simulink model "test_sys2"  (R2013b)
settings: Solver=ode45  StartTime=0.0  StopTime=5000  RelTol=1e-3
undefined symbols (not defined in the file or in its folder): twiddle_factors, xlipgetpartsetting
libraries: xbsIndex_r4 x2526, casper_library_misc x201, xps_library x1
(part 1 of 29)
settings Model: Creator=root  LastModifiedBy=root

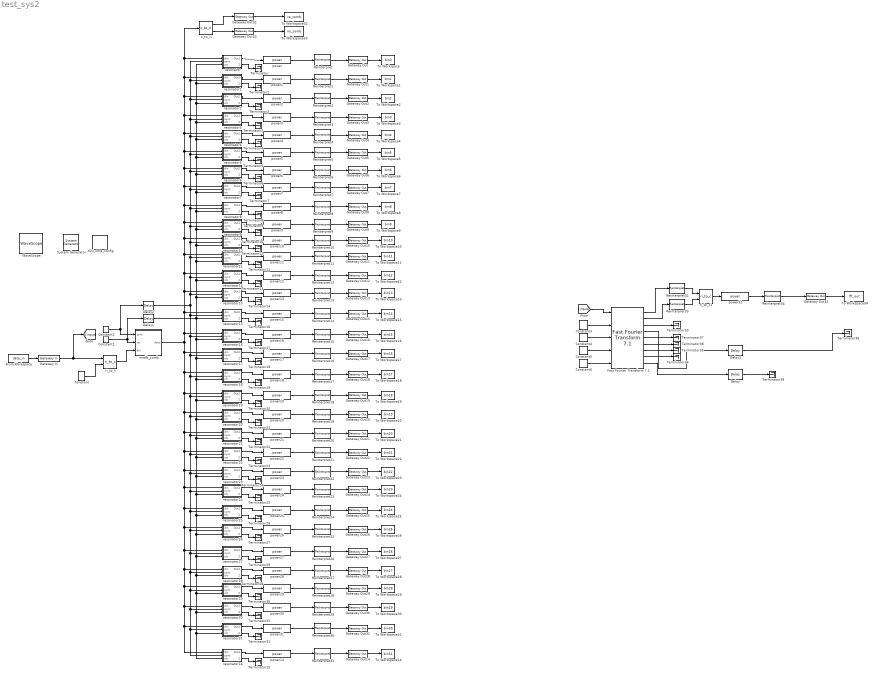
== system test_sys2 ==
  " System Generator" : xbsIndex_r4/ System Generator  Tag=genX  xilinxfamily=Kintex7  part=xc7k325t  speed=-3  package=fbg676  synthesis_tool=XST  clock_wrapper=Clock Enables  directory=./netlist  proj_type=Project Navigator  Synth_file=XST Defaults  Impl_file=ISE Defaults  testbench=off  simulink_period=1  sysclk_period=10  dcm_input_clock_period=10  incr_netlist=off  trim_vbits=Everywhere in SubSystem  dbl_ovrd=According to Block Masks  core_generation=According to Block Masks  run_coregen=off  deprecated_control=off  eval_field=0  block_type=sysgen
  Constant : xbsIndex_r4/Constant  const=0  gui_display_data_type=Fixed-point  arith_type=Signed (2's comp)  n_bits=10  bin_pt=9  preci_type=Single  exp_width=8  frac_width=24  explicit_period=on  period=1  equ=P=C  opselect=C  inp2=PCIN>>17  opr=+  inp1=P  carry=CIN  dbl_ovrd=off  block_type=constant
  Constant1 : xbsIndex_r4/Constant  const=0  gui_display_data_type=Boolean  arith_type=Boolean  n_bits=16  bin_pt=14  preci_type=Single  exp_width=8  frac_width=24  explicit_period=on  period=1  equ=P=C  opselect=C  inp2=PCIN>>17  opr=+  inp1=P  carry=CIN  dbl_ovrd=off  block_type=constant
  Constant2 : xbsIndex_r4/Constant  const=1  gui_display_data_type=Boolean  arith_type=Boolean  n_bits=16  bin_pt=14  preci_type=Single  exp_width=8  frac_width=24  explicit_period=on  period=1  equ=P=C  opselect=C  inp2=PCIN>>17  opr=+  inp1=P  carry=CIN  dbl_ovrd=off  block_type=constant
  Constant3 : xbsIndex_r4/Constant  const=0  gui_display_data_type=Fixed-point  arith_type=Signed (2's comp)  n_bits=10  bin_pt=9  preci_type=Single  exp_width=8  frac_width=24  explicit_period=on  period=1  equ=P=C  opselect=C  inp2=PCIN>>17  opr=+  inp1=P  carry=CIN  dbl_ovrd=off  block_type=constant
  Constant4 : xbsIndex_r4/Constant  const=1  gui_display_data_type=Boolean  arith_type=Boolean  n_bits=10  bin_pt=9  preci_type=Single  exp_width=8  frac_width=24  explicit_period=on  period=1  equ=P=C  opselect=C  inp2=PCIN>>17  opr=+  inp1=P  carry=CIN  dbl_ovrd=off  block_type=constant
  Constant5 : xbsIndex_r4/Constant  const=1  gui_display_data_type=Boolean  arith_type=Boolean  n_bits=10  bin_pt=9  preci_type=Single  exp_width=8  frac_width=24  explicit_period=on  period=1  equ=P=C  opselect=C  inp2=PCIN>>17  opr=+  inp1=P  carry=CIN  dbl_ovrd=off  block_type=constant
  Constant6 : xbsIndex_r4/Constant  const=0  gui_display_data_type=Boolean  arith_type=Boolean  n_bits=10  bin_pt=9  preci_type=Single  exp_width=8  frac_width=24  explicit_period=on  period=1  equ=P=C  opselect=C  inp2=PCIN>>17  opr=+  inp1=P  carry=CIN  dbl_ovrd=off  block_type=constant
  Delay : xbsIndex_r4/Delay  rst=off  infoeditControl=Selection of Reset will increase slice count due to use of real FFs and instead of SRLs  en=off  latency=5  dbl_ovrd=off  reg_retiming=off  block_type=delay
  Delay1 : xbsIndex_r4/Delay  rst=off  infoeditControl=Selection of Reset will increase slice count due to use of real FFs and instead of SRLs  en=off  latency=1  dbl_ovrd=off  reg_retiming=off  block_type=delay
  Delay2 : xbsIndex_r4/Delay  rst=off  infoeditControl=Selection of Reset will increase slice count due to use of real FFs and instead of SRLs  en=off  latency=1  dbl_ovrd=off  reg_retiming=off  block_type=delay
  Delay3 : xbsIndex_r4/Delay  rst=off  infoeditControl=Selection of Reset will increase slice count due to use of real FFs and instead of SRLs  en=off  latency=5  dbl_ovrd=off  reg_retiming=off  block_type=delay
  "Fast Fourier Transform 7.1 " : xbsIndex_r4/Fast Fourier Transform 7.1   transform_length=128  implementation_options=pipelined_streaming_io  target_clock_frequency=250  target_data_throughput=50  run_time_configurable_transform_length=off  phase_factor_width=16  scaling_options=unscaled  rounding_modes=convergent_rounding  output_ordering=natural_order  cyclic_prefix_insertion=off  ce=off  sclr=off  ovflo=off  input_data_offset=three_cycle_offset  memory_options_data=block_ram  memory_options_phase_factors=block_ram  number_of_stages_using_block_ram_for_data_and_phase_factors=1  memory_options_reorder=block_ram  memory_options_hybrid=off  complex_mult_type=use_mults_performance  butterfly_type=use_luts  channels=1  input_ordering=natural_order  input_width=16  simulation_type=external_xfix  simulation_model=fftv71_CModel:fftv71_cmodel  ip_name=Fast Fourier Transform  ip_version=7.1  dsptool_ready=true  wrapper_available=true  port_translation_map={ 'ce' => 'en', 'sclr' => 'rst' }  ipcore_fpga_part=xlipgetpartsetting(gcb, {'virtex4', 'xc4vsx35', '-10', 'ff668'})  block_type=xfft_v7_1
  From Workspace : FromWorkspace  VariableName=data_in  SampleTime=0
  Gateway In : xbsIndex_r4/Gateway In  gui_display_data_type=Fixed-point  arith_type="Signed  (2's comp)"  n_bits=10  bin_pt=9  preci_type=Single  exp_width=8  frac_width=24  quantization="Round  (unbiased: +/- Inf)"  overflow=Saturate  period=1  dbl_ovrd=off  timing_constraint=None  locs_specified=off  LOCs={}  UseAsADC=off  ADCChannel='1'  inherit_from_input=off  hdl_port=on  block_type=gatewayin
  Gateway Out{,1..34} (35 alike) : xbsIndex_r4/Gateway Out  inherit_from_input=off  hdl_port=on  timing_constraint=None  locs_specified=off  LOCs={}  UseAsDAC=off  DACChannel='1'  block_type=gatewayout
  Reinterpret{,1..31,34} (33 alike) : xbsIndex_r4/Reinterpret  force_arith_type=off  arith_type=Unsigned  force_bin_pt=on  bin_pt=0  block_type=reinterpret
  Reinterpret32 : xbsIndex_r4/Reinterpret  force_arith_type=off  arith_type=Unsigned  force_bin_pt=on  bin_pt=17  block_type=reinterpret
  Reinterpret33 : xbsIndex_r4/Reinterpret  force_arith_type=off  arith_type=Unsigned  force_bin_pt=on  bin_pt=17  block_type=reinterpret
  Terminator{,1..39} (40 alike) : Terminator
  To Workspace : ToWorkspace  VariableName=bin0  SampleTime=-1  SaveFormat=Timeseries
  To Workspace1 : ToWorkspace  VariableName=bin1  SampleTime=-1  SaveFormat=Timeseries
  To Workspace10 : ToWorkspace  VariableName=bin10  SampleTime=-1  SaveFormat=Timeseries
  To Workspace11 : ToWorkspace  VariableName=bin11  SampleTime=-1  SaveFormat=Timeseries
  To Workspace12 : ToWorkspace  VariableName=bin12  SampleTime=-1  SaveFormat=Timeseries
  To Workspace13 : ToWorkspace  VariableName=bin13  SampleTime=-1  SaveFormat=Timeseries
  To Workspace14 : ToWorkspace  VariableName=bin31  SampleTime=-1  SaveFormat=Timeseries
  To Workspace15 : ToWorkspace  VariableName=bin14  SampleTime=-1  SaveFormat=Timeseries
  To Workspace16 : ToWorkspace  VariableName=bin15  SampleTime=-1  SaveFormat=Timeseries
  To Workspace17 : ToWorkspace  VariableName=bin16  SampleTime=-1  SaveFormat=Timeseries
  To Workspace18 : ToWorkspace  VariableName=bin17  SampleTime=-1  SaveFormat=Timeseries
  To Workspace19 : ToWorkspace  VariableName=bin18  SampleTime=-1  SaveFormat=Timeseries
  To Workspace2 : ToWorkspace  VariableName=bin2  SampleTime=-1  SaveFormat=Timeseries
  To Workspace20 : ToWorkspace  VariableName=bin19  SampleTime=-1  SaveFormat=Timeseries
  To Workspace21 : ToWorkspace  VariableName=bin20  SampleTime=-1  SaveFormat=Timeseries
  To Workspace22 : ToWorkspace  VariableName=bin21  SampleTime=-1  SaveFormat=Timeseries
  To Workspace23 : ToWorkspace  VariableName=bin22  SampleTime=-1  SaveFormat=Timeseries
  To Workspace24 : ToWorkspace  VariableName=bin23  SampleTime=-1  SaveFormat=Timeseries
  To Workspace25 : ToWorkspace  VariableName=bin24  SampleTime=-1  SaveFormat=Timeseries
  To Workspace26 : ToWorkspace  VariableName=bin25  SampleTime=-1  SaveFormat=Timeseries
  To Workspace27 : ToWorkspace  VariableName=bin26  SampleTime=-1  SaveFormat=Timeseries
  To Workspace28 : ToWorkspace  VariableName=bin27  SampleTime=-1  SaveFormat=Timeseries
  To Workspace29 : ToWorkspace  VariableName=bin28  SampleTime=-1  SaveFormat=Timeseries
  To Workspace3 : ToWorkspace  VariableName=bin3  SampleTime=-1  SaveFormat=Timeseries
  To Workspace30 : ToWorkspace  VariableName=bin29  SampleTime=-1  SaveFormat=Timeseries
  To Workspace31 : ToWorkspace  VariableName=bin30  SampleTime=-1  SaveFormat=Timeseries
  To Workspace32 : ToWorkspace  VariableName=re_comb  SampleTime=-1  SaveFormat=Timeseries
  To Workspace33 : ToWorkspace  VariableName=im_comb  SampleTime=-1  SaveFormat=Timeseries
  To Workspace34 : ToWorkspace  VariableName=fft_out  SampleTime=-1  SaveFormat=Timeseries
  To Workspace4 : ToWorkspace  VariableName=bin4  SampleTime=-1  SaveFormat=Timeseries
  To Workspace5 : ToWorkspace  VariableName=bin5  SampleTime=-1  SaveFormat=Timeseries
  To Workspace6 : ToWorkspace  VariableName=bin6  SampleTime=-1  SaveFormat=Timeseries
  To Workspace7 : ToWorkspace  VariableName=bin7  SampleTime=-1  SaveFormat=Timeseries
  To Workspace8 : ToWorkspace  VariableName=bin8  SampleTime=-1  SaveFormat=Timeseries
  To Workspace9 : ToWorkspace  VariableName=bin9  SampleTime=-1  SaveFormat=Timeseries
  WaveScope : xbsIndex_r4/WaveScope  block_type=wavescope
  XSG_core_config : xps_library/XSG_core_config  Tag=xps:xsg  hw_sys=ROACH2:sx475t  clk_src=sys_clk  ROACH_clk_src=sys_clk  ROACH2_clk_src=sys_clk  MKDIG_clk_src=sys_clk  clk_rate=100  sample_period=1  synthesis_tool=XST
  c_to_ri : casper_library_misc/c_to_ri  n_bits=11  bin_pt=9
      settings: AttributesFormatString=11_9 r/i
  msdft_comb : Subsystem  mask(msdft_comb){input_bitsize=10, fft_len=7, latency=0}
      mask prompts: fft_len "fft_len (2^?)"; latency "sub latency"
      mask init:
      | msdft_comb_init(gcb, ...
      |         'input_bitsize', input_bitsize, ...
      |         'fft_len', fft_len, ...
      |         'latency', latency);
      settings: AttributesFormatString=latency=0
  power{,1..31} (32 alike) : casper_library_misc/power  BitWidth=40  add_latency=2  mult_latency=3
  power32 : casper_library_misc/power  BitWidth=18  add_latency=2  mult_latency=3
  resonator : Subsystem  mask(msdft_res){fft_len=7, twid_bitsize=15, bin_number=0, input_bitsize=11, input_frac=9, res_bitsize=40, add_lat=0}
      mask prompts: fft_len "fft len(2^?)"; twid_bitsize "twid bitsize"; bin_number "bin number"; input_bitsize "input bitsize"; input_frac "input frac"; res_bitsize "out resonator size"
      mask init:
      | msdft_resonator_init(gcb, ...
      |                 'fft_len', fft_len, ...
      |                 'twid_bitsize', twid_bitsize, ...
      |                 'bin_number', bin_number, ...
      |                 'input_bitsize', input_bitsize, ...
      |                 'input_frac', input_frac, ...
      |                 'res_bitsize', res_bitsize, ...
      |                 'add_lat', add_lat);
      settings: AttributesFormatString=N=7, k=0
  resonator1 : Subsystem  mask(msdft_res){fft_len=7, twid_bitsize=15, bin_number=1, input_bitsize=11, input_frac=9, res_bitsize=40, add_lat=0}
      mask prompts: fft_len "fft len(2^?)"; twid_bitsize "twid bitsize"; bin_number "bin number"; input_bitsize "input bitsize"; input_frac "input frac"; res_bitsize "out resonator size"
      mask init: same as test_sys2/resonator
      settings: AttributesFormatString=N=7, k=1
  resonator10 : Subsystem  mask(msdft_res){fft_len=7, twid_bitsize=15, bin_number=10, input_bitsize=11, input_frac=9, res_bitsize=40, add_lat=0}
      mask prompts: fft_len "fft len(2^?)"; twid_bitsize "twid bitsize"; bin_number "bin number"; input_bitsize "input bitsize"; input_frac "input frac"; res_bitsize "out resonator size"
      mask init: same as test_sys2/resonator
      settings: AttributesFormatString=N=7, k=10
  resonator11 : Subsystem  mask(msdft_res){fft_len=7, twid_bitsize=15, bin_number=11, input_bitsize=11, input_frac=9, res_bitsize=40, add_lat=0}
      mask prompts: fft_len "fft len(2^?)"; twid_bitsize "twid bitsize"; bin_number "bin number"; input_bitsize "input bitsize"; input_frac "input frac"; res_bitsize "out resonator size"
      mask init: same as test_sys2/resonator
      settings: AttributesFormatString=N=7, k=11
  resonator12 : Subsystem  mask(msdft_res){fft_len=7, twid_bitsize=15, bin_number=12, input_bitsize=11, input_frac=9, res_bitsize=40, add_lat=0}
      mask prompts: fft_len "fft len(2^?)"; twid_bitsize "twid bitsize"; bin_number "bin number"; input_bitsize "input bitsize"; input_frac "input frac"; res_bitsize "out resonator size"
      mask init: same as test_sys2/resonator
      settings: AttributesFormatString=N=7, k=12
  resonator13 : Subsystem  mask(msdft_res){fft_len=7, twid_bitsize=15, bin_number=13, input_bitsize=11, input_frac=9, res_bitsize=40, add_lat=0}
      mask prompts: fft_len "fft len(2^?)"; twid_bitsize "twid bitsize"; bin_number "bin number"; input_bitsize "input bitsize"; input_frac "input frac"; res_bitsize "out resonator size"
      mask init: same as test_sys2/resonator
      settings: AttributesFormatString=N=7, k=13
  resonator14 : Subsystem  mask(msdft_res){fft_len=7, twid_bitsize=15, bin_number=31, input_bitsize=11, input_frac=9, res_bitsize=40, add_lat=0}
      mask prompts: fft_len "fft len(2^?)"; twid_bitsize "twid bitsize"; bin_number "bin number"; input_bitsize "input bitsize"; input_frac "input frac"; res_bitsize "out resonator size"
      mask init: same as test_sys2/resonator
      settings: AttributesFormatString=N=7, k=31
  resonator15 : Subsystem  mask(msdft_res){fft_len=7, twid_bitsize=15, bin_number=14, input_bitsize=11, input_frac=9, res_bitsize=40, add_lat=0}
      mask prompts: fft_len "fft len(2^?)"; twid_bitsize "twid bitsize"; bin_number "bin number"; input_bitsize "input bitsize"; input_frac "input frac"; res_bitsize "out resonator size"
      mask init: same as test_sys2/resonator
      settings: AttributesFormatString=N=7, k=14
  resonator16 : Subsystem  mask(msdft_res){fft_len=7, twid_bitsize=15, bin_number=15, input_bitsize=11, input_frac=9, res_bitsize=40, add_lat=0}
      mask prompts: fft_len "fft len(2^?)"; twid_bitsize "twid bitsize"; bin_number "bin number"; input_bitsize "input bitsize"; input_frac "input frac"; res_bitsize "out resonator size"
      mask init: same as test_sys2/resonator
      settings: AttributesFormatString=N=7, k=15
  resonator17 : Subsystem  mask(msdft_res){fft_len=7, twid_bitsize=15, bin_number=16, input_bitsize=11, input_frac=9, res_bitsize=40, add_lat=0}
      mask prompts: fft_len "fft len(2^?)"; twid_bitsize "twid bitsize"; bin_number "bin number"; input_bitsize "input bitsize"; input_frac "input frac"; res_bitsize "out resonator size"
      mask init: same as test_sys2/resonator
      settings: AttributesFormatString=N=7, k=16
  resonator18 : Subsystem  mask(msdft_res){fft_len=7, twid_bitsize=15, bin_number=17, input_bitsize=11, input_frac=9, res_bitsize=40, add_lat=0}
      mask prompts: fft_len "fft len(2^?)"; twid_bitsize "twid bitsize"; bin_number "bin number"; input_bitsize "input bitsize"; input_frac "input frac"; res_bitsize "out resonator size"
      mask init: same as test_sys2/resonator
      settings: AttributesFormatString=N=7, k=17
  resonator19 : Subsystem  mask(msdft_res){fft_len=7, twid_bitsize=15, bin_number=18, input_bitsize=11, input_frac=9, res_bitsize=40, add_lat=0}
      mask prompts: fft_len "fft len(2^?)"; twid_bitsize "twid bitsize"; bin_number "bin number"; input_bitsize "input bitsize"; input_frac "input frac"; res_bitsize "out resonator size"
      mask init: same as test_sys2/resonator
      settings: AttributesFormatString=N=7, k=18
  resonator2 : Subsystem  mask(msdft_res){fft_len=7, twid_bitsize=15, bin_number=2, input_bitsize=11, input_frac=9, res_bitsize=40, add_lat=0}
      mask prompts: fft_len "fft len(2^?)"; twid_bitsize "twid bitsize"; bin_number "bin number"; input_bitsize "input bitsize"; input_frac "input frac"; res_bitsize "out resonator size"
      mask init: same as test_sys2/resonator
      settings: AttributesFormatString=N=7, k=2
  resonator20 : Subsystem  mask(msdft_res){fft_len=7, twid_bitsize=15, bin_number=19, input_bitsize=11, input_frac=9, res_bitsize=40, add_lat=0}
      mask prompts: fft_len "fft len(2^?)"; twid_bitsize "twid bitsize"; bin_number "bin number"; input_bitsize "input bitsize"; input_frac "input frac"; res_bitsize "out resonator size"
      mask init: same as test_sys2/resonator
      settings: AttributesFormatString=N=7, k=19
  resonator21 : Subsystem  mask(msdft_res){fft_len=7, twid_bitsize=15, bin_number=20, input_bitsize=11, input_frac=9, res_bitsize=40, add_lat=0}
      mask prompts: fft_len "fft len(2^?)"; twid_bitsize "twid bitsize"; bin_number "bin number"; input_bitsize "input bitsize"; input_frac "input frac"; res_bitsize "out resonator size"
      mask init: same as test_sys2/resonator
      settings: AttributesFormatString=N=7, k=20
  resonator22 : Subsystem  mask(msdft_res){fft_len=7, twid_bitsize=15, bin_number=21, input_bitsize=11, input_frac=9, res_bitsize=40, add_lat=0}
      mask prompts: fft_len "fft len(2^?)"; twid_bitsize "twid bitsize"; bin_number "bin number"; input_bitsize "input bitsize"; input_frac "input frac"; res_bitsize "out resonator size"
      mask init: same as test_sys2/resonator
      settings: AttributesFormatString=N=7, k=21
  resonator23 : Subsystem  mask(msdft_res){fft_len=7, twid_bitsize=15, bin_number=22, input_bitsize=11, input_frac=9, res_bitsize=40, add_lat=0}
      mask prompts: fft_len "fft len(2^?)"; twid_bitsize "twid bitsize"; bin_number "bin number"; input_bitsize "input bitsize"; input_frac "input frac"; res_bitsize "out resonator size"
      mask init: same as test_sys2/resonator
      settings: AttributesFormatString=N=7, k=22
  resonator24 : Subsystem  mask(msdft_res){fft_len=7, twid_bitsize=15, bin_number=23, input_bitsize=11, input_frac=9, res_bitsize=40, add_lat=0}
      mask prompts: fft_len "fft len(2^?)"; twid_bitsize "twid bitsize"; bin_number "bin number"; input_bitsize "input bitsize"; input_frac "input frac"; res_bitsize "out resonator size"
      mask init: same as test_sys2/resonator
      settings: AttributesFormatString=N=7, k=23
  resonator25 : Subsystem  mask(msdft_res){fft_len=7, twid_bitsize=15, bin_number=24, input_bitsize=11, input_frac=9, res_bitsize=40, add_lat=0}
      mask prompts: fft_len "fft len(2^?)"; twid_bitsize "twid bitsize"; bin_number "bin number"; input_bitsize "input bitsize"; input_frac "input frac"; res_bitsize "out resonator size"
      mask init: same as test_sys2/resonator
      settings: AttributesFormatString=N=7, k=24
  resonator26 : Subsystem  mask(msdft_res){fft_len=7, twid_bitsize=15, bin_number=25, input_bitsize=11, input_frac=9, res_bitsize=40, add_lat=0}
      mask prompts: fft_len "fft len(2^?)"; twid_bitsize "twid bitsize"; bin_number "bin number"; input_bitsize "input bitsize"; input_frac "input frac"; res_bitsize "out resonator size"
      mask init: same as test_sys2/resonator
      settings: AttributesFormatString=N=7, k=25
  resonator27 : Subsystem  mask(msdft_res){fft_len=7, twid_bitsize=15, bin_number=26, input_bitsize=11, input_frac=9, res_bitsize=40, add_lat=0}
      mask prompts: fft_len "fft len(2^?)"; twid_bitsize "twid bitsize"; bin_number "bin number"; input_bitsize "input bitsize"; input_frac "input frac"; res_bitsize "out resonator size"
      mask init: same as test_sys2/resonator
      settings: AttributesFormatString=N=7, k=26
  resonator28 : Subsystem  mask(msdft_res){fft_len=7, twid_bitsize=15, bin_number=27, input_bitsize=11, input_frac=9, res_bitsize=40, add_lat=0}
      mask prompts: fft_len "fft len(2^?)"; twid_bitsize "twid bitsize"; bin_number "bin number"; input_bitsize "input bitsize"; input_frac "input frac"; res_bitsize "out resonator size"
      mask init: same as test_sys2/resonator
      settings: AttributesFormatString=N=7, k=27
  resonator29 : Subsystem  mask(msdft_res){fft_len=7, twid_bitsize=15, bin_number=28, input_bitsize=11, input_frac=9, res_bitsize=40, add_lat=0}
      mask prompts: fft_len "fft len(2^?)"; twid_bitsize "twid bitsize"; bin_number "bin number"; input_bitsize "input bitsize"; input_frac "input frac"; res_bitsize "out resonator size"
      mask init: same as test_sys2/resonator
      settings: AttributesFormatString=N=7, k=28
  resonator3 : Subsystem  mask(msdft_res){fft_len=7, twid_bitsize=15, bin_number=3, input_bitsize=11, input_frac=9, res_bitsize=40, add_lat=0}
      mask prompts: fft_len "fft len(2^?)"; twid_bitsize "twid bitsize"; bin_number "bin number"; input_bitsize "input bitsize"; input_frac "input frac"; res_bitsize "out resonator size"
      mask init: same as test_sys2/resonator
      settings: AttributesFormatString=N=7, k=3
  resonator30 : Subsystem  mask(msdft_res){fft_len=7, twid_bitsize=15, bin_number=29, input_bitsize=11, input_frac=9, res_bitsize=40, add_lat=0}
      mask prompts: fft_len "fft len(2^?)"; twid_bitsize "twid bitsize"; bin_number "bin number"; input_bitsize "input bitsize"; input_frac "input frac"; res_bitsize "out resonator size"
      mask init: same as test_sys2/resonator
      settings: AttributesFormatString=N=7, k=29
  resonator31 : Subsystem  mask(msdft_res){fft_len=7, twid_bitsize=15, bin_number=30, input_bitsize=11, input_frac=9, res_bitsize=40, add_lat=0}
      mask prompts: fft_len "fft len(2^?)"; twid_bitsize "twid bitsize"; bin_number "bin number"; input_bitsize "input bitsize"; input_frac "input frac"; res_bitsize "out resonator size"
      mask init: same as test_sys2/resonator
      settings: AttributesFormatString=N=7, k=30
  resonator4 : Subsystem  mask(msdft_res){fft_len=7, twid_bitsize=15, bin_number=4, input_bitsize=11, input_frac=9, res_bitsize=40, add_lat=0}
      mask prompts: fft_len "fft len(2^?)"; twid_bitsize "twid bitsize"; bin_number "bin number"; input_bitsize "input bitsize"; input_frac "input frac"; res_bitsize "out resonator size"
      mask init: same as test_sys2/resonator
      settings: AttributesFormatString=N=7, k=4
  resonator5 : Subsystem  mask(msdft_res){fft_len=7, twid_bitsize=15, bin_number=5, input_bitsize=11, input_frac=9, res_bitsize=40, add_lat=0}
      mask prompts: fft_len "fft len(2^?)"; twid_bitsize "twid bitsize"; bin_number "bin number"; input_bitsize "input bitsize"; input_frac "input frac"; res_bitsize "out resonator size"
      mask init: same as test_sys2/resonator
      settings: AttributesFormatString=N=7, k=5
  resonator6 : Subsystem  mask(msdft_res){fft_len=7, twid_bitsize=15, bin_number=6, input_bitsize=11, input_frac=9, res_bitsize=40, add_lat=0}
      mask prompts: fft_len "fft len(2^?)"; twid_bitsize "twid bitsize"; bin_number "bin number"; input_bitsize "input bitsize"; input_frac "input frac"; res_bitsize "out resonator size"
      mask init: same as test_sys2/resonator
      settings: AttributesFormatString=N=7, k=6
  resonator7 : Subsystem  mask(msdft_res){fft_len=7, twid_bitsize=15, bin_number=7, input_bitsize=11, input_frac=9, res_bitsize=40, add_lat=0}
      mask prompts: fft_len "fft len(2^?)"; twid_bitsize "twid bitsize"; bin_number "bin number"; input_bitsize "input bitsize"; input_frac "input frac"; res_bitsize "out resonator size"
      mask init: same as test_sys2/resonator
      settings: AttributesFormatString=N=7, k=7
  resonator8 : Subsystem  mask(msdft_res){fft_len=7, twid_bitsize=15, bin_number=8, input_bitsize=11, input_frac=9, res_bitsize=40, add_lat=0}
      mask prompts: fft_len "fft len(2^?)"; twid_bitsize "twid bitsize"; bin_number "bin number"; input_bitsize "input bitsize"; input_frac "input frac"; res_bitsize "out resonator size"
      mask init: same as test_sys2/resonator
      settings: AttributesFormatString=N=7, k=8
  resonator9 : Subsystem  mask(msdft_res){fft_len=7, twid_bitsize=15, bin_number=9, input_bitsize=11, input_frac=9, res_bitsize=40, add_lat=0}
      mask prompts: fft_len "fft len(2^?)"; twid_bitsize "twid bitsize"; bin_number "bin number"; input_bitsize "input bitsize"; input_frac "input frac"; res_bitsize "out resonator size"
      mask init: same as test_sys2/resonator
      settings: AttributesFormatString=N=7, k=9
  ri_to_c : casper_library_misc/ri_to_c
  ri_to_c1 : casper_library_misc/ri_to_c
  wires:
  Constant1/1 -> Delay1/1, msdft_comb/2(rst)
  resonator/1(Out1) -> power/1
  resonator/2(twidd) -> Terminator/1
  power/1 -> Reinterpret/1
  Gateway Out/1 -> To Workspace/1
  From Workspace/1 -> Gateway In/1
  resonator1/1(Out1) -> power1/1
  resonator1/2(twidd) -> Terminator1/1
  power1/1 -> Reinterpret1/1
  Gateway Out1/1 -> To Workspace1/1
  resonator2/1(Out1) -> power2/1
  resonator2/2(twidd) -> Terminator2/1
  power2/1 -> Reinterpret2/1
  Gateway Out2/1 -> To Workspace2/1
  resonator3/2(twidd) -> Terminator3/1
  power3/1 -> Reinterpret3/1
  resonator3/1(Out1) -> power3/1
  Gateway Out3/1 -> To Workspace3/1
  resonator4/2(twidd) -> Terminator4/1
  power4/1 -> Reinterpret4/1
  resonator4/1(Out1) -> power4/1
  Gateway Out4/1 -> To Workspace4/1
  resonator5/2(twidd) -> Terminator5/1
  resonator5/1(Out1) -> power5/1
  power5/1 -> Reinterpret5/1
  Gateway Out5/1 -> To Workspace5/1
  resonator6/2(twidd) -> Terminator6/1
  resonator6/1(Out1) -> power6/1
  power6/1 -> Reinterpret6/1
  Gateway Out6/1 -> To Workspace6/1
  resonator7/2(twidd) -> Terminator7/1
  resonator7/1(Out1) -> power7/1
  power7/1 -> Reinterpret7/1
  Gateway Out7/1 -> To Workspace7/1
  resonator8/2(twidd) -> Terminator8/1
  resonator8/1(Out1) -> power8/1
  power8/1 -> Reinterpret8/1
  Gateway Out8/1 -> To Workspace8/1
  resonator9/2(twidd) -> Terminator9/1
  resonator9/1(Out1) -> power9/1
  power9/1 -> Reinterpret9/1
  Gateway Out9/1 -> To Workspace9/1
  resonator10/2(twidd) -> Terminator10/1
  resonator10/1(Out1) -> power10/1
  power10/1 -> Reinterpret10/1
  Gateway Out10/1 -> To Workspace10/1
  msdft_comb/1(dout) -> resonator16/1(din), resonator13/1(din), resonator12/1(din), resonator11/1(din), resonator10/1(din), resonator9/1(din), resonator5/1(din), resonator4/1(din), resonator2/1(din), resonator1/1(din), c_to_ri/1, resonator/1(din), resonator3/1(din), resonator6/1(din), resonator7/1(din), resonator8/1(din), resonator15/1(din), resonator17/1(din), resonator18/1(din), resonator19/1(din), resonator21/1(din), resonator23/1(din), resonator24/1(din), resonator25/1(din), resonator27/1(din), resonator28/1(din), resonator29/1(din), resonator31/1(din), resonator14/1(din), resonator30/1(din), resonator26/1(din), resonator22/1(din), resonator20/1(din)
  Delay2/1 -> resonator17/2(sync), resonator21/2(sync), resonator31/2(sync), resonator14/2(sync), resonator30/2(sync), resonator29/2(sync), resonator28/2(sync), resonator27/2(sync), resonator26/2(sync), resonator25/2(sync), resonator24/2(sync), resonator23/2(sync), resonator22/2(sync), resonator20/2(sync), resonator19/2(sync), resonator18/2(sync), resonator16/2(sync), resonator15/2(sync), resonator13/2(sync), resonator12/2(sync), resonator11/2(sync), resonator10/2(sync), resonator9/2(sync), resonator6/2(sync), resonator5/2(sync), resonator4/2(sync), resonator3/2(sync), resonator2/2(sync), resonator1/2(sync), resonator/2(sync), resonator7/2(sync), resonator8/2(sync)
  Delay1/1 -> resonator15/3(rst), resonator18/3(rst), resonator25/3(rst), resonator28/3(rst), resonator29/3(rst), resonator30/3(rst), resonator14/3(rst), resonator31/3(rst), resonator27/3(rst), resonator26/3(rst), resonator24/3(rst), resonator23/3(rst), resonator22/3(rst), resonator21/3(rst), resonator20/3(rst), resonator19/3(rst), resonator17/3(rst), resonator16/3(rst), resonator13/3(rst), resonator12/3(rst), resonator11/3(rst), resonator10/3(rst), resonator9/3(rst), resonator8/3(rst), resonator6/3(rst), resonator5/3(rst), resonator4/3(rst), resonator3/3(rst), resonator2/3(rst), resonator1/3(rst), resonator/3(rst), resonator7/3(rst)
  resonator11/2(twidd) -> Terminator11/1
  resonator11/1(Out1) -> power11/1
  power11/1 -> Reinterpret11/1
  Gateway Out11/1 -> To Workspace11/1
  resonator12/2(twidd) -> Terminator13/1
  resonator12/1(Out1) -> power12/1
  power12/1 -> Reinterpret12/1
  Gateway Out12/1 -> To Workspace12/1
  resonator13/2(twidd) -> Terminator14/1
  resonator13/1(Out1) -> power13/1
  power13/1 -> Reinterpret13/1
  Gateway Out13/1 -> To Workspace13/1
  resonator14/2(twidd) -> Terminator15/1
  resonator14/1(Out1) -> power14/1
  power14/1 -> Reinterpret31/1
  Gateway Out14/1 -> To Workspace14/1
  resonator15/2(twidd) -> Terminator16/1
  resonator15/1(Out1) -> power15/1
  power15/1 -> Reinterpret14/1
  Gateway Out15/1 -> To Workspace15/1
  resonator16/2(twidd) -> Terminator17/1
  resonator16/1(Out1) -> power16/1
  power16/1 -> Reinterpret15/1
  Gateway Out16/1 -> To Workspace16/1
  resonator17/2(twidd) -> Terminator18/1
  resonator17/1(Out1) -> power17/1
  power17/1 -> Reinterpret16/1
  Gateway Out17/1 -> To Workspace17/1
  resonator18/2(twidd) -> Terminator19/1
  resonator18/1(Out1) -> power18/1
  power18/1 -> Reinterpret17/1
  Gateway Out18/1 -> To Workspace18/1
  resonator19/2(twidd) -> Terminator20/1
  resonator19/1(Out1) -> power19/1
  power19/1 -> Reinterpret18/1
  Gateway Out19/1 -> To Workspace19/1
  resonator20/2(twidd) -> Terminator21/1
  resonator20/1(Out1) -> power20/1
  power20/1 -> Reinterpret19/1
  Gateway Out20/1 -> To Workspace20/1
  resonator21/2(twidd) -> Terminator22/1
  resonator21/1(Out1) -> power21/1
  power21/1 -> Reinterpret20/1
  Gateway Out21/1 -> To Workspace21/1
  resonator22/2(twidd) -> Terminator23/1
  resonator22/1(Out1) -> power22/1
  power22/1 -> Reinterpret21/1
  Gateway Out22/1 -> To Workspace22/1
  resonator23/2(twidd) -> Terminator24/1
  resonator23/1(Out1) -> power23/1
  power23/1 -> Reinterpret22/1
  Gateway Out23/1 -> To Workspace23/1
  resonator24/2(twidd) -> Terminator25/1
  resonator24/1(Out1) -> power24/1
  power24/1 -> Reinterpret23/1
  Gateway Out24/1 -> To Workspace24/1
  resonator25/2(twidd) -> Terminator26/1
  resonator25/1(Out1) -> power25/1
  power25/1 -> Reinterpret24/1
  Gateway Out25/1 -> To Workspace25/1
  resonator26/2(twidd) -> Terminator27/1
  resonator26/1(Out1) -> power26/1
  power26/1 -> Reinterpret25/1
  Gateway Out26/1 -> To Workspace26/1
  resonator27/2(twidd) -> Terminator29/1
  resonator27/1(Out1) -> power27/1
  power27/1 -> Reinterpret26/1
  Gateway Out27/1 -> To Workspace27/1
  resonator28/2(twidd) -> Terminator28/1
  resonator28/1(Out1) -> power28/1
  power28/1 -> Reinterpret27/1
  Gateway Out28/1 -> To Workspace28/1
  resonator29/2(twidd) -> Terminator30/1
  resonator29/1(Out1) -> power29/1
  power29/1 -> Reinterpret28/1
  Gateway Out29/1 -> To Workspace29/1
  resonator30/2(twidd) -> Terminator32/1
  resonator30/1(Out1) -> power30/1
  power30/1 -> Reinterpret29/1
  Gateway Out30/1 -> To Workspace30/1
  resonator31/2(twidd) -> Terminator31/1
  resonator31/1(Out1) -> power31/1
  power31/1 -> Reinterpret30/1
  Gateway Out31/1 -> To Workspace31/1
  Gateway In/1 -> [input], ri_to_c/1
  Constant/1 -> ri_to_c/2
  ri_to_c/1 -> msdft_comb/3(din)
  Constant2/1 -> Delay2/1, msdft_comb/1(sync)
  c_to_ri/1 -> Gateway Out32/1
  c_to_ri/2 -> Gateway Out33/1
  Gateway Out32/1 -> To Workspace32/1
  Gateway Out33/1 -> To Workspace33/1
  Reinterpret/1 -> Gateway Out/1
  Reinterpret1/1 -> Gateway Out1/1
  Reinterpret2/1 -> Gateway Out2/1
  Reinterpret3/1 -> Gateway Out3/1
  Reinterpret4/1 -> Gateway Out4/1
  Reinterpret5/1 -> Gateway Out5/1
  Reinterpret6/1 -> Gateway Out6/1
  Reinterpret7/1 -> Gateway Out7/1
  Reinterpret8/1 -> Gateway Out8/1
  Reinterpret9/1 -> Gateway Out9/1
  Reinterpret10/1 -> Gateway Out10/1
  Reinterpret11/1 -> Gateway Out11/1
  Reinterpret12/1 -> Gateway Out12/1
  Reinterpret13/1 -> Gateway Out13/1
  Reinterpret14/1 -> Gateway Out15/1
  Reinterpret15/1 -> Gateway Out16/1
  Reinterpret16/1 -> Gateway Out17/1
  Reinterpret17/1 -> Gateway Out18/1
  Reinterpret18/1 -> Gateway Out19/1
  Reinterpret19/1 -> Gateway Out20/1
  Reinterpret20/1 -> Gateway Out21/1
  Reinterpret21/1 -> Gateway Out22/1
  Reinterpret22/1 -> Gateway Out23/1
  Reinterpret23/1 -> Gateway Out24/1
  Reinterpret24/1 -> Gateway Out25/1
  Reinterpret25/1 -> Gateway Out26/1
  Reinterpret26/1 -> Gateway Out27/1
  Reinterpret27/1 -> Gateway Out28/1
  Reinterpret28/1 -> Gateway Out29/1
  Reinterpret29/1 -> Gateway Out30/1
  Reinterpret30/1 -> Gateway Out31/1
  Reinterpret31/1 -> Gateway Out14/1
  [input] -> "Fast Fourier Transform 7.1 "/1
  Constant3/1 -> "Fast Fourier Transform 7.1 "/2
  Constant4/1 -> "Fast Fourier Transform 7.1 "/3
  Constant5/1 -> "Fast Fourier Transform 7.1 "/4
  Constant6/1 -> "Fast Fourier Transform 7.1 "/5
  "Fast Fourier Transform 7.1 "/1 -> Reinterpret32/1
  "Fast Fourier Transform 7.1 "/2 -> Reinterpret33/1
  "Fast Fourier Transform 7.1 "/8 -> Terminator34/1
  "Fast Fourier Transform 7.1 "/7 -> Terminator35/1
  "Fast Fourier Transform 7.1 "/3 -> Terminator33/1
  "Fast Fourier Transform 7.1 "/4 -> Delay3/1
  "Fast Fourier Transform 7.1 "/5 -> Terminator37/1
  "Fast Fourier Transform 7.1 "/6 -> Terminator38/1
  Reinterpret32/1 -> ri_to_c1/1
  Reinterpret33/1 -> ri_to_c1/2
  ri_to_c1/1 -> power32/1
  power32/1 -> Reinterpret34/1
  Gateway Out34/1 -> To Workspace34/1
  "Fast Fourier Transform 7.1 "/9 -> Delay/1
  Delay/1 -> Terminator39/1
  Reinterpret34/1 -> Gateway Out34/1
  Delay3/1 -> Terminator36/1

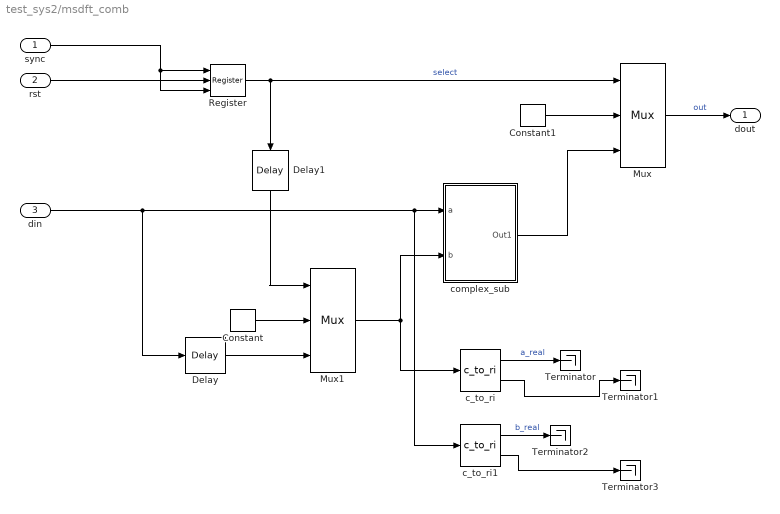
== system test_sys2/msdft_comb ==
  sync : Inport
  rst : Inport  Port=2
  din : Inport  Port=3
  Constant : xbsIndex_r4/Constant  const=0  gui_display_data_type=Fixed-point  arith_type=Unsigned  n_bits=2*input_bitsize  bin_pt=0  preci_type=Single  exp_width=8  frac_width=24  explicit_period=on  period=1  equ=P=C  opselect=C  inp2=PCIN>>17  opr=+  inp1=P  carry=CIN  dbl_ovrd=off  block_type=constant
  Constant1 : xbsIndex_r4/Constant  const=0  gui_display_data_type=Fixed-point  arith_type=Unsigned  n_bits=2*(input_bitsize+1)  bin_pt=0  preci_type=Single  exp_width=8  frac_width=24  explicit_period=on  period=1  equ=P=C  opselect=C  inp2=PCIN>>17  opr=+  inp1=P  carry=CIN  dbl_ovrd=off  block_type=constant
  Delay : xbsIndex_r4/Delay  rst=off  infoeditControl=Selection of Reset will increase slice count due to use of real FFs and instead of SRLs  en=off  latency=2^fft_len  dbl_ovrd=off  reg_retiming=off  block_type=delay
  Delay1 : xbsIndex_r4/Delay  rst=off  infoeditControl=Selection of Reset will increase slice count due to use of real FFs and instead of SRLs  en=off  latency=2^fft_len-1  dbl_ovrd=off  reg_retiming=off  block_type=delay
  Mux : xbsIndex_r4/Mux  inputs=2  en=off  latency=0  precision=Full  arith_type=Unsigned  n_bits=16  bin_pt=14  quantization=Truncate  overflow=Wrap  dbl_ovrd=off  block_type=mux
  Mux1 : xbsIndex_r4/Mux  inputs=2  en=off  latency=0  precision=Full  arith_type=Unsigned  n_bits=16  bin_pt=14  quantization=Truncate  overflow=Wrap  dbl_ovrd=off  block_type=mux
  Register : xbsIndex_r4/Register  init=0  rst=on  en=on  dbl_ovrd=off  block_type=register
  Terminator{,1..3} (4 alike) : Terminator
  c_to_ri : casper_library_misc/c_to_ri  n_bits=10  bin_pt=9
      settings: AttributesFormatString=10_9 r/i
  c_to_ri1 : casper_library_misc/c_to_ri  n_bits=10  bin_pt=9
      settings: AttributesFormatString=10_9 r/i
  complex_sub : Subsystem  mask(complex_sub){a_bitsize=input_bitsize, b_bitsize=input_bitsize, latency=0}
      mask init:
      | complex_sub_init(gcb, ...
      |             'a_bitsize', a_bitsize, ...
      |             'b_bitsize', b_bitsize, ...
      |             'latency', latency);
      settings: AttributesFormatString=latency=0
  dout : Outport
  wires:
  sync/1 -> Register/3, Register/1
  rst/1 -> Register/2
  din/1 -> Delay/1, c_to_ri1/1, complex_sub/1("a ")
  complex_sub/1(Out1) -> Mux/3
  Delay/1 -> Mux1/3
  Constant/1 -> Mux1/2
  Constant1/1 -> Mux/2
  Mux1/1 -> complex_sub/2(b), c_to_ri/1
  Mux/1 -> dout/1  "out"
  Register/1 -> Mux/1, Delay1/1  "select"
  c_to_ri/1 -> Terminator/1  "a_real"
  c_to_ri/2 -> Terminator1/1
  c_to_ri1/1 -> Terminator2/1  "b_real"
  c_to_ri1/2 -> Terminator3/1
  Delay1/1 -> Mux1/1

== system test_sys2/resonator ==
  note: No estoy tan seguro
      | de este delay....
  din : Inport
  sync : Inport  Port=2
  rst : Inport  Port=3
  Delay{,1..2,4} (4 alike) : xbsIndex_r4/Delay  rst=off  infoeditControl=Selection of Reset will increase slice count due to use of real FFs and instead of SRLs  en=off  latency=1  dbl_ovrd=off  reg_retiming=off  block_type=delay
  Delay3 : xbsIndex_r4/Delay  rst=off  infoeditControl=Selection of Reset will increase slice count due to use of real FFs and instead of SRLs  en=off  latency=5  dbl_ovrd=off  reg_retiming=off  block_type=delay
  cmult : Subsystem  AncestorBlock=casper_library_multipliers/cmult  mask(cmult){n_bits_a=input_bitsize, bin_pt_a=input_frac, n_bits_b=twid_bitsize, bin_pt_b=twid_bitsize-2, n_bits_ab=input_bitsize+twid_bitsize+1, bin_pt_ab=input_frac+twid_bitsize-2, quantization=Truncate, overflow=Wrap, in_latency=0, mult_latency=3, add_latency=1, conv_latency=1, conjugated=off, async=off, pipelined_enable=on, multiplier_implementation=behavioral HDL}
      mask prompts: n_bits_a "Number of Bits 'a'"; bin_pt_a "Binary Point 'a'"; n_bits_b "Number of Bits 'b'"; bin_pt_b "Binary Point 'b'"; n_bits_ab "Number of Bits 'ab'"; bin_pt_ab "Binary Point 'ab'"; in_latency "Input latency"; mult_latency "Multiplier Latency"; add_latency "Adder Latency"; conv_latency "Convert latency"; conjugated "Conjugate"; async "asynchronous operation"; pipelined_enable "enable pipeline"; multiplier_implementation "Multiplier implementation"
      mask help:
      | Multiplies two complex numbers using 4 multipliers and 2 adders.
      | Conjugation is optional.
      mask init:
      | cmult_init(gcb, ...
      |     'n_bits_a',n_bits_a, ...
      |     'bin_pt_a',bin_pt_a, ...
      |     'n_bits_b',n_bits_b, ...
      |     'bin_pt_b',bin_pt_b, ...
      |     'n_bits_ab',n_bits_ab, ...
      |     'bin_pt_ab',bin_pt_ab, ...
      |     'quantization',quantization, ...
      |     'overflow', overflow, ...
      |     'in_latency', in_latency, ...
      |     'mult_latency', mult_latency, ...
      |     'add_latency', add_latency, ...
      |     'conv_latency', conv_latency, ...
      |     'conjugated', conjugated, ...
      |     'multiplier_implementation', multiplier_implementation, ...
      |     'async', async, ...
      |     'pipelined_enable', pipelined_enable);
      settings: AttributesFormatString=|
      | 11_9 * 15_13 ==> 27_22
      | Truncate, Wrap
      | Latency=0
      mask TypeOptions quantization: Truncate | Round  (unbiased: +/- Inf) | Round  (unbiased: Even Values)
      mask TypeOptions overflow: Wrap | Saturate | Flag as error
      mask TypeOptions multiplier_implementation: behavioral HDL | standard core | embedded multiplier core
  complex_conj : Subsystem  AncestorBlock=casper_library_misc/complex_conj  mask(complex_conj){n_inputs=1, n_bits=twid_bitsize, bin_pt=twid_bitsize-2, latency=1, overflow=Wrap}
      mask prompts: n_inputs "number simultaneous inputs"; n_bits "input bitwidth"; bin_pt "input binary point"; overflow "overflow strategy"
      mask help: Finds the complex conjugate of complex inputs.
      mask init:
      | complex_conj_init(gcb, ...
      |     'n_inputs', n_inputs, ...
      |     'n_bits', n_bits, ...
      |     'bin_pt', bin_pt, ...
      |     'latency', latency, ...
      |     'overflow', overflow);
      mask TypeOptions overflow: Wrap | Saturate | Flag as error
  complex_sum : Subsystem  mask(complex_sum){a_bitsize=input_bitsize+twid_bitsize+1, a_frac=input_frac+twid_bitsize-2, b_bitsize=res_bitsize, b_frac=input_frac+twid_bitsize-2, out_bitsize=res_bitsize, latency=add_lat}
      mask prompts: out_bitsize "output_bitsize"
      mask init:
      | complex_sum_init(gcb, ...
      |             'a_bitsize', a_bitsize, ...
      |             'a_frac', a_frac, ...
      |             'b_bitsize', b_bitsize, ...
      |             'b_frac', b_frac, ...
      |             'out_bitsize', out_bitsize, ...
      |             'latency', latency);
      settings: AttributesFormatString=latency=0
  twiddle : Subsystem  mask(msdft_twiddle_factors){fft_len=fft_len, bin_num=bin_number, twid_bitsize=twid_bitsize}
      mask prompts: fft_len "fft_len(2^)"; bin_num "bin number"; twid_bitsize "twiddle bitsize"
      mask init:
      | twid_msdft_init(gcb, ...
      |         'fft_len', fft_len, ...
      |         'bin_num', bin_num, ...
      |         'twid_bitsize', twid_bitsize)
      settings: AttributesFormatString=N=7, k=0
  Out1 : Outport
  twidd : Outport  Port=2
  wires:
  sync/1 -> twiddle/1(sync)
  rst/1 -> twiddle/2(rst)
  din/1 -> Delay/1
  twiddle/1(dout) -> complex_conj/1(z), Delay1/1
  complex_conj/1(z*) -> cmult/2(b)
  Delay/1 -> cmult/1(a)
  cmult/1(ab) -> complex_sum/1(a)
  complex_sum/1(dout) -> Delay2/1, Out1/1
  Delay2/1 -> complex_sum/2(b)
  Delay1/1 -> Delay3/1
  Delay3/1 -> Delay4/1
  Delay4/1 -> twidd/1

== system test_sys2/resonator1 ==
  note: No estoy tan seguro
      | de este delay....
  din : Inport
  sync : Inport  Port=2
  rst : Inport  Port=3
  Delay{,1..2,4} (4 alike) : xbsIndex_r4/Delay  rst=off  infoeditControl=Selection of Reset will increase slice count due to use of real FFs and instead of SRLs  en=off  latency=1  dbl_ovrd=off  reg_retiming=off  block_type=delay
  Delay3 : xbsIndex_r4/Delay  rst=off  infoeditControl=Selection of Reset will increase slice count due to use of real FFs and instead of SRLs  en=off  latency=5  dbl_ovrd=off  reg_retiming=off  block_type=delay
  cmult : Subsystem  AncestorBlock=casper_library_multipliers/cmult  mask(cmult){n_bits_a=input_bitsize, bin_pt_a=input_frac, n_bits_b=twid_bitsize, bin_pt_b=twid_bitsize-2, n_bits_ab=input_bitsize+twid_bitsize+1, bin_pt_ab=input_frac+twid_bitsize-2, quantization=Truncate, overflow=Wrap, in_latency=0, mult_latency=3, add_latency=1, conv_latency=1, conjugated=off, async=off, pipelined_enable=on, multiplier_implementation=behavioral HDL}
      mask prompts: n_bits_a "Number of Bits 'a'"; bin_pt_a "Binary Point 'a'"; n_bits_b "Number of Bits 'b'"; bin_pt_b "Binary Point 'b'"; n_bits_ab "Number of Bits 'ab'"; bin_pt_ab "Binary Point 'ab'"; in_latency "Input latency"; mult_latency "Multiplier Latency"; add_latency "Adder Latency"; conv_latency "Convert latency"; conjugated "Conjugate"; async "asynchronous operation"; pipelined_enable "enable pipeline"; multiplier_implementation "Multiplier implementation"
      mask help:
      | Multiplies two complex numbers using 4 multipliers and 2 adders.
      | Conjugation is optional.
      mask init: same as test_sys2/resonator/cmult
      settings: AttributesFormatString=|
      | 11_9 * 15_13 ==> 27_22
      | Truncate, Wrap
      | Latency=0
      mask TypeOptions quantization: Truncate | Round  (unbiased: +/- Inf) | Round  (unbiased: Even Values)
      mask TypeOptions overflow: Wrap | Saturate | Flag as error
      mask TypeOptions multiplier_implementation: behavioral HDL | standard core | embedded multiplier core
  complex_conj : Subsystem  AncestorBlock=casper_library_misc/complex_conj  mask(complex_conj){n_inputs=1, n_bits=twid_bitsize, bin_pt=twid_bitsize-2, latency=1, overflow=Wrap}
      mask prompts: n_inputs "number simultaneous inputs"; n_bits "input bitwidth"; bin_pt "input binary point"; overflow "overflow strategy"
      mask help: Finds the complex conjugate of complex inputs.
      mask init:
      | complex_conj_init(gcb, ...
      |     'n_inputs', n_inputs, ...
      |     'n_bits', n_bits, ...
      |     'bin_pt', bin_pt, ...
      |     'latency', latency, ...
      |     'overflow', overflow);
      mask TypeOptions overflow: Wrap | Saturate | Flag as error
  complex_sum : Subsystem  mask(complex_sum){a_bitsize=input_bitsize+twid_bitsize+1, a_frac=input_frac+twid_bitsize-2, b_bitsize=res_bitsize, b_frac=input_frac+twid_bitsize-2, out_bitsize=res_bitsize, latency=add_lat}
      mask prompts: out_bitsize "output_bitsize"
      mask init: same as test_sys2/resonator/complex_sum
      settings: AttributesFormatString=latency=0
  twiddle : Subsystem  mask(msdft_twiddle_factors){fft_len=fft_len, bin_num=bin_number, twid_bitsize=twid_bitsize}
      mask prompts: fft_len "fft_len(2^)"; bin_num "bin number"; twid_bitsize "twiddle bitsize"
      mask init:
      | twid_msdft_init(gcb, ...
      |         'fft_len', fft_len, ...
      |         'bin_num', bin_num, ...
      |         'twid_bitsize', twid_bitsize)
      settings: AttributesFormatString=N=7, k=1
  Out1 : Outport
  twidd : Outport  Port=2
  wires:
  sync/1 -> twiddle/1(sync)
  rst/1 -> twiddle/2(rst)
  din/1 -> Delay/1
  twiddle/1(dout) -> complex_conj/1(z), Delay1/1
  complex_conj/1(z*) -> cmult/2(b)
  Delay/1 -> cmult/1(a)
  cmult/1(ab) -> complex_sum/1(a)
  complex_sum/1(dout) -> Delay2/1, Out1/1
  Delay2/1 -> complex_sum/2(b)
  Delay1/1 -> Delay3/1
  Delay3/1 -> Delay4/1
  Delay4/1 -> twidd/1

== system test_sys2/resonator10 ==
  note: No estoy tan seguro
      | de este delay....
  din : Inport
  sync : Inport  Port=2
  rst : Inport  Port=3
  Delay{,1..2,4} (4 alike) : xbsIndex_r4/Delay  rst=off  infoeditControl=Selection of Reset will increase slice count due to use of real FFs and instead of SRLs  en=off  latency=1  dbl_ovrd=off  reg_retiming=off  block_type=delay
  Delay3 : xbsIndex_r4/Delay  rst=off  infoeditControl=Selection of Reset will increase slice count due to use of real FFs and instead of SRLs  en=off  latency=5  dbl_ovrd=off  reg_retiming=off  block_type=delay
  cmult : Subsystem  AncestorBlock=casper_library_multipliers/cmult  mask(cmult){n_bits_a=input_bitsize, bin_pt_a=input_frac, n_bits_b=twid_bitsize, bin_pt_b=twid_bitsize-2, n_bits_ab=input_bitsize+twid_bitsize+1, bin_pt_ab=input_frac+twid_bitsize-2, quantization=Truncate, overflow=Wrap, in_latency=0, mult_latency=3, add_latency=1, conv_latency=1, conjugated=off, async=off, pipelined_enable=on, multiplier_implementation=behavioral HDL}
      mask prompts: n_bits_a "Number of Bits 'a'"; bin_pt_a "Binary Point 'a'"; n_bits_b "Number of Bits 'b'"; bin_pt_b "Binary Point 'b'"; n_bits_ab "Number of Bits 'ab'"; bin_pt_ab "Binary Point 'ab'"; in_latency "Input latency"; mult_latency "Multiplier Latency"; add_latency "Adder Latency"; conv_latency "Convert latency"; conjugated "Conjugate"; async "asynchronous operation"; pipelined_enable "enable pipeline"; multiplier_implementation "Multiplier implementation"
      mask help:
      | Multiplies two complex numbers using 4 multipliers and 2 adders.
      | Conjugation is optional.
      mask init: same as test_sys2/resonator/cmult
      settings: AttributesFormatString=|
      | 11_9 * 15_13 ==> 27_22
      | Truncate, Wrap
      | Latency=0
      mask TypeOptions quantization: Truncate | Round  (unbiased: +/- Inf) | Round  (unbiased: Even Values)
      mask TypeOptions overflow: Wrap | Saturate | Flag as error
      mask TypeOptions multiplier_implementation: behavioral HDL | standard core | embedded multiplier core
  complex_conj : Subsystem  AncestorBlock=casper_library_misc/complex_conj  mask(complex_conj){n_inputs=1, n_bits=twid_bitsize, bin_pt=twid_bitsize-2, latency=1, overflow=Wrap}
      mask prompts: n_inputs "number simultaneous inputs"; n_bits "input bitwidth"; bin_pt "input binary point"; overflow "overflow strategy"
      mask help: Finds the complex conjugate of complex inputs.
      mask init:
      | complex_conj_init(gcb, ...
      |     'n_inputs', n_inputs, ...
      |     'n_bits', n_bits, ...
      |     'bin_pt', bin_pt, ...
      |     'latency', latency, ...
      |     'overflow', overflow);
      mask TypeOptions overflow: Wrap | Saturate | Flag as error
  complex_sum : Subsystem  mask(complex_sum){a_bitsize=input_bitsize+twid_bitsize+1, a_frac=input_frac+twid_bitsize-2, b_bitsize=res_bitsize, b_frac=input_frac+twid_bitsize-2, out_bitsize=res_bitsize, latency=add_lat}
      mask prompts: out_bitsize "output_bitsize"
      mask init: same as test_sys2/resonator/complex_sum
      settings: AttributesFormatString=latency=0
  twiddle : Subsystem  mask(msdft_twiddle_factors){fft_len=fft_len, bin_num=bin_number, twid_bitsize=twid_bitsize}
      mask prompts: fft_len "fft_len(2^)"; bin_num "bin number"; twid_bitsize "twiddle bitsize"
      mask init:
      | twid_msdft_init(gcb, ...
      |         'fft_len', fft_len, ...
      |         'bin_num', bin_num, ...
      |         'twid_bitsize', twid_bitsize)
      settings: AttributesFormatString=N=7, k=10
  Out1 : Outport
  twidd : Outport  Port=2
  wires:
  sync/1 -> twiddle/1(sync)
  rst/1 -> twiddle/2(rst)
  din/1 -> Delay/1
  twiddle/1(dout) -> complex_conj/1(z), Delay1/1
  complex_conj/1(z*) -> cmult/2(b)
  Delay/1 -> cmult/1(a)
  cmult/1(ab) -> complex_sum/1(a)
  complex_sum/1(dout) -> Delay2/1, Out1/1
  Delay2/1 -> complex_sum/2(b)
  Delay1/1 -> Delay3/1
  Delay3/1 -> Delay4/1
  Delay4/1 -> twidd/1
